simulink model "SYSTEME_ZIGBEE"  (R2016b)
settings: Solver=ode45  StartTime=0.0  StopTime=1E-3  RelTol=1e-3
libraries: dspsrcs4 x6, dsparch4 x5, simulink x3, dspstat3 x2, commsink2 x1, commrandsrc2 x1, commdigbbndcpm2 x1, dspsigops x1
settings Model: DisableUpgradeWarningsForVersion=R2015a  Creator=Yannis  LastModifiedBy=root
settings DataIOCC: LimitDataPoints=on  SaveFormat=Array
settings OptimizationCC: BlockReduction=off  BooleanDataType=off  LifeSpan=inf
settings DebuggingCC: SaveWithParameterizedLinksMsg=none  UnderspecifiedInitializationDetection=Classic  MergeDetectMultiDrivingBlocksExec=none  SignalResolutionControl=TryResolveAllWithWarning  SFUnexpectedBacktrackingDiag=warning  SFNoUnconditionalDefaultTransitionDiag=warning  SFExecutionAtInitializationDiag=none
settings HardwareCC: ProdBitPerPointer=32  ProdBitPerSizeT=32  ProdBitPerPtrDiffT=32  ProdLargestAtomicFloat=None  ProdIntDivRoundTo=Undefined  ProdEndianess=Unspecified  ProdWordSize=32  ProdHWDeviceType=32-bit Generic  TargetBitPerLong=64  TargetBitPerPointer=64  TargetBitPerSizeT=64  TargetBitPerPtrDiffT=64  TargetLongLongMode=on  TargetIntDivRoundTo=Zero  TargetEndianess=LittleEndian  TargetWordSize=64  TargetHWDeviceType=MATLAB Host  ProdEqTarget=off
settings ModelReferenceCC: PropagateSignalLabelsOutOfModel=off
settings GRTTargetCC: TargetLangStandard=C89/C90 (ANSI)  GeneratePreprocessorConditionals=Disable all
settings ConfigComp: CovMetricSettings=dw  CovHtmlReporting=on  CovSaveCumulativeToWorkspaceVar=on  CovSaveSingleToWorkspaceVar=on  CovExternalEMLEnable=off

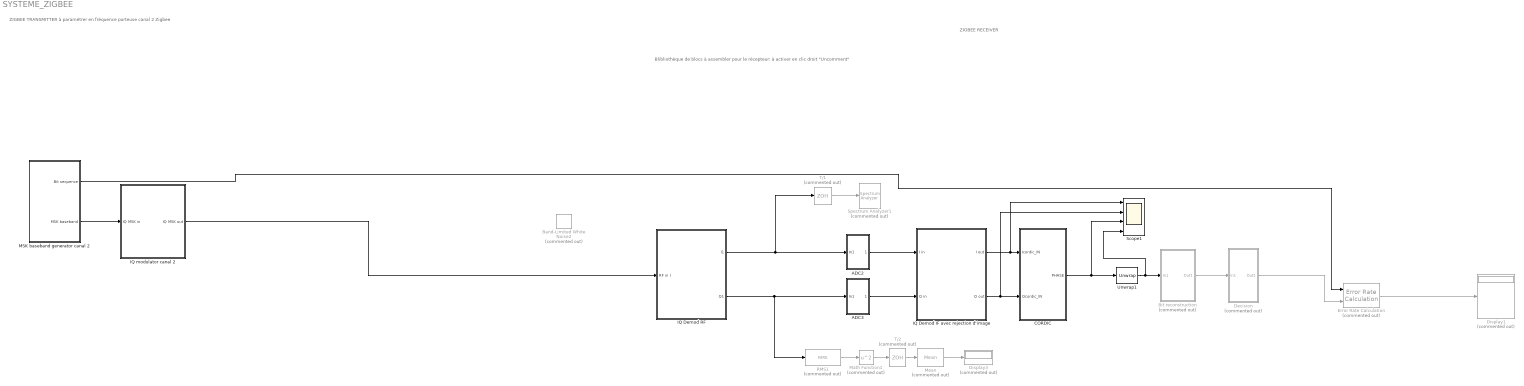
== system SYSTEME_ZIGBEE ==
  note: ZIGBEE RECEIVER
  note: ZIGBEE TRANSMITTER
      | à paramétrer en fréquence porteuse
      | canal 2  Zigbee
  note: Blibliothèque de blocs à assembler pour le récepteur: à activer en clic droit "Uncomment"
  ADC2 : Subsystem
  ADC3 : Subsystem
  Band-Limited White Noise2 : simulink/Sources/Band-Limited White Noise  Commented=on  Cov=[1e-7]  Ts=1e-10  seed=[23341]
  Bit reconstruction : Subsystem  Commented=on
  CORDIC : Subsystem
  Decision : Subsystem  Commented=on
  Display1 : Display  Commented=on
  Display3 : Display  Commented=on
  Error Rate Calculation : commsink2/Error Rate Calculation  Commented=on  N=2  st_delay=1  cp_mode=Entire frame  subframe=[]  PMode=Port  WsName=ErrorVec  RsMode2=off  stop=off  numErr=100  maxBits=1e6
  IQ Demod IF avec rejection d'image : Subsystem  TreatAsAtomicUnit=on
  IQ Demod RF : Subsystem  TreatAsAtomicUnit=on
  IQ modulator canal 2 : Subsystem
  MSK baseband generator canal 2 : Subsystem
  Math Function1 : Math  Commented=on  Operator=square  SaturateOnIntegerOverflow=on
  Mean : dspstat3/Mean  Commented=on  run=on  reset_popup=None  InputProcessing=Columns as channels (frame based)  directionMode=Each column  dimension=1  roiEnable=off  roiType=Rectangles  roiPortion=Entire ROI  roiOutput=Individual statistics for each ROI  roiFlag=off  outputDataTypeStr=Inherit: Same as accumulator  outputLastDataTypeStr=Inherit: Same as accumulator  outputMin=[]  outputMax=[]  roundingMode=Floor  overflowMode=off
  RMS1 : dspstat3/RMS  Commented=on  run=off  directionMode=Entire input  dimension=1  InputProcessing=Columns as channels (frame based)  reset_popup=None
  Scope1 : Scope  NumInputPorts=4
  Spectrum Analyzer1 : SpectrumAnalyzer  Commented=on
  T/1 : ZeroOrderHold  Commented=on  SampleTime=1/(10e6)
  T/2 : ZeroOrderHold  Commented=on  SampleTime=1/(10e6)
  Unwrap1 : dspsigops/Unwrap  tol=pi  InputProcessing=Columns as channels (frame based)  running=off
  wires:
  MSK baseband generator canal 2/2(MSK baseband) -> IQ modulator canal 2/1(IQ MSK in)
  MSK baseband generator canal 2/1(Bit sequence) -> Error Rate Calculation/1
  Error Rate Calculation/1 -> Display1/1
  ADC2/1(Out1) -> IQ Demod IF avec rejection d'image/1("I in ")
  ADC3/1(Out1) -> IQ Demod IF avec rejection d'image/2("Q in ")
  IQ Demod RF/1(I1) -> T/1/1, ADC2/1(In1)
  IQ Demod RF/2("Q1 ") -> RMS1/1, ADC3/1(In1)
  IQ Demod IF avec rejection d'image/1(I out) -> Scope1/1, CORDIC/1(Icordic_IN)
  IQ Demod IF avec rejection d'image/2(Q out) -> Scope1/2, CORDIC/2(Qcordic_IN)
  CORDIC/1(PHASE) -> Scope1/3, Unwrap1/1
  Unwrap1/1 -> Scope1/4, Bit reconstruction/1(In1)
  Bit reconstruction/1(Out1) -> Decision/1(In1)
  T/1/1 -> Spectrum Analyzer1/1
  Decision/1(Out1) -> Error Rate Calculation/2
  RMS1/1 -> Math Function1/1
  Math Function1/1 -> T/2/1
  Mean/1 -> Display3/1
  T/2/1 -> Mean/1
  IQ modulator canal 2/1("IQ MSK out ") -> IQ Demod RF/1(RF in I)

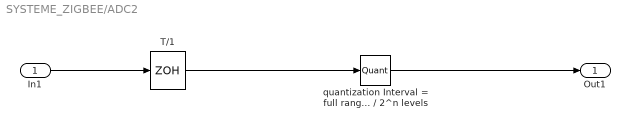
== system SYSTEME_ZIGBEE/ADC2 ==
  In1 : Inport
  T/1 : ZeroOrderHold  SampleTime=1/(10e6)
  quantization Interval = full range (2Volts) / 2^n levels : Quantizer  QuantizationInterval=2/256  LinearizeAsGain=off  SampleTime=1/(10e6)
  Out1 : Outport
  wires:
  In1/1 -> T/1/1
  T/1/1 -> quantization Interval = full range (2Volts) / 2^n levels/1
  quantization Interval = full range (2Volts) / 2^n levels/1 -> Out1/1

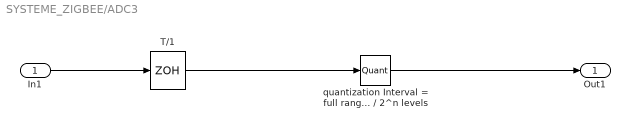
== system SYSTEME_ZIGBEE/ADC3 ==
  In1 : Inport
  T/1 : ZeroOrderHold  SampleTime=1/(10e6)
  quantization Interval = full range (2Volts) / 2^n levels : Quantizer  QuantizationInterval=2/256  LinearizeAsGain=off  SampleTime=1/(10e6)
  Out1 : Outport
  wires:
  In1/1 -> T/1/1
  T/1/1 -> quantization Interval = full range (2Volts) / 2^n levels/1
  quantization Interval = full range (2Volts) / 2^n levels/1 -> Out1/1

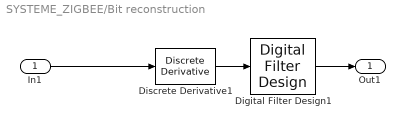
== system SYSTEME_ZIGBEE/Bit reconstruction ==
  In1 : Inport
  Digital Filter Design1 : dsparch4/Digital Filter Design  mwdsp_browser_bugfix_var=off
  Discrete Derivative1 : simulink/Discrete/Discrete Derivative  gainval=1/(10e6)  ICPrevScaledInput=0.0  InputProcessing=Inherited  OutMin=[]  OutMax=[]  OutDataTypeStr=double  OutputDataTypeScalingMode=double  OutDataType=fixdt(1, 16)  OutScaling=2^-10  DoSatur=off
  Out1 : Outport
  wires:
  Discrete Derivative1/1 -> Digital Filter Design1/1
  Digital Filter Design1/1 -> Out1/1
  In1/1 -> Discrete Derivative1/1

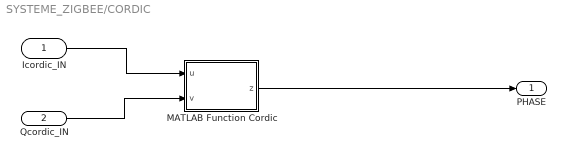
== system SYSTEME_ZIGBEE/CORDIC ==
  Icordic_IN : Inport
  Qcordic_IN : Inport  Port=2
  MATLAB Function Cordic : MATLAB Function  TreatAsAtomicUnit=on
  PHASE : Outport
  wires:
  MATLAB Function Cordic/1(z) -> PHASE/1
  Icordic_IN/1 -> MATLAB Function Cordic/1(u)
  Qcordic_IN/1 -> MATLAB Function Cordic/2(v)

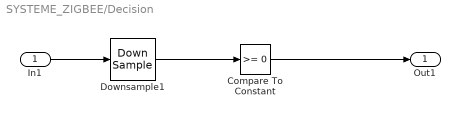
== system SYSTEME_ZIGBEE/Decision ==
  In1 : Inport
  Compare To Constant : simulink/Logic and Bit Operations/Compare To Constant  relop=>=  const=0  OutDataTypeStr=boolean
  Downsample1 : DownSample  N=5  phase=2
  Out1 : Outport
  wires:
  Compare To Constant/1 -> Out1/1
  In1/1 -> Downsample1/1
  Downsample1/1 -> Compare To Constant/1

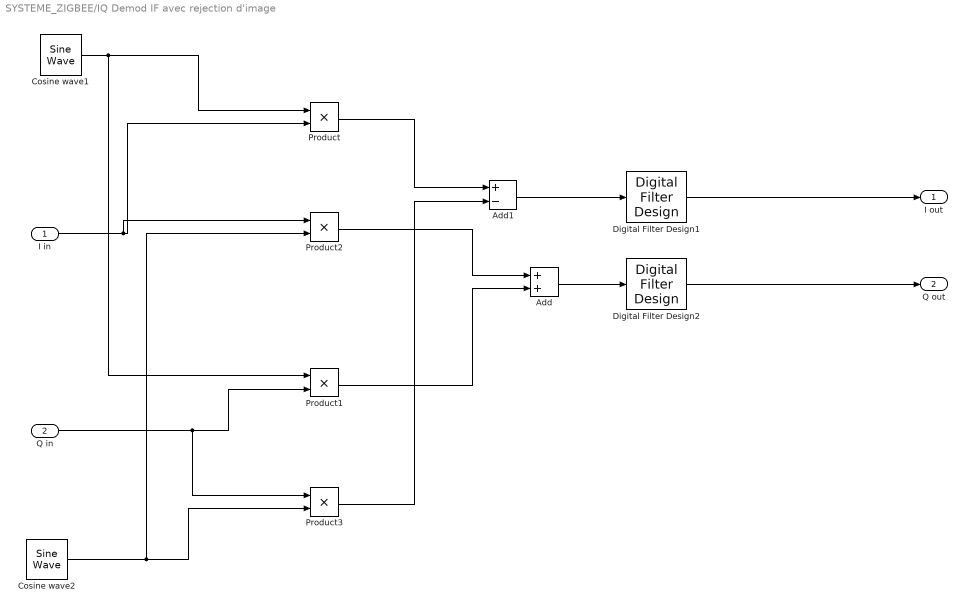
== system SYSTEME_ZIGBEE/IQ Demod IF avec rejection d'image ==
  "I in " : Inport
  "Q in " : Inport  Port=2
  Add : Sum
  Add1 : Sum  Inputs=+-
  Cosine wave1 : dspsrcs4/Sine Wave  Amplitude=1  Frequency=2.5e6  Phase=pi/2  SampleMode=Discrete  OutComplex=Real  CompMethod=Trigonometric fcn  TableSize=Speed  SampleTime=1/(10e6)  SamplesPerFrame=1  ResetState=Restart at time zero  OutputFrames=on  dataType=double  wordLen=16  udDataType=sfix(16)  fracBitsMode=Best precision  numFracBits=15  OutDataTypeStr=double  LastOutDataTypeStr=double
  Cosine wave2 : dspsrcs4/Sine Wave  Amplitude=1  Frequency=2.5e6  Phase=pi  SampleMode=Discrete  OutComplex=Real  CompMethod=Trigonometric fcn  TableSize=Speed  SampleTime=1/(10e6)  SamplesPerFrame=1  ResetState=Restart at time zero  OutputFrames=on  dataType=double  wordLen=16  udDataType=sfix(16)  fracBitsMode=Best precision  numFracBits=15  OutDataTypeStr=double  LastOutDataTypeStr=double
  Digital Filter Design1 : dsparch4/Digital Filter Design  mwdsp_browser_bugfix_var=off
  Digital Filter Design2 : dsparch4/Digital Filter Design  mwdsp_browser_bugfix_var=off
  Product{,1..3} (4 alike) : Product
  I out : Outport
  Q out : Outport  Port=2
  wires:
  Digital Filter Design1/1 -> I out/1
  Digital Filter Design2/1 -> Q out/1
  Cosine wave1/1 -> Product1/1, Product/1
  Cosine wave2/1 -> Product2/2, Product3/2
  "I in "/1 -> Product2/1, Product/2
  "Q in "/1 -> Product3/1, Product1/2
  Product/1 -> Add1/1
  Product3/1 -> Add1/2
  Product2/1 -> Add/1
  Product1/1 -> Add/2
  Add/1 -> Digital Filter Design2/1
  Add1/1 -> Digital Filter Design1/1

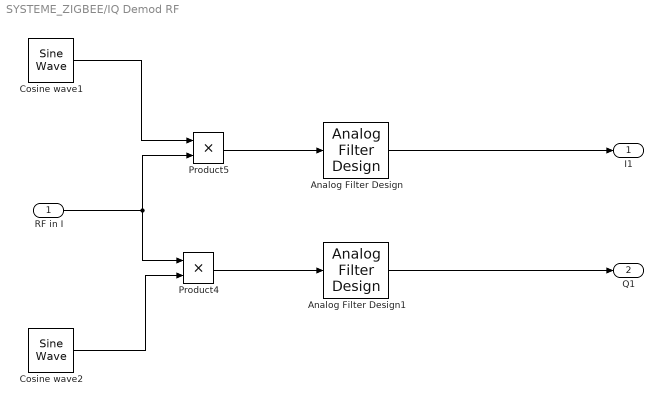
== system SYSTEME_ZIGBEE/IQ Demod RF ==
  RF in I : Inport
  Analog Filter Design : dsparch4/Analog Filter Design  method=Butterworth  filttype=Lowpass  N=8  Wlo=31.4e6  Whi=80  Rp=2  Rs=40
  Analog Filter Design1 : dsparch4/Analog Filter Design  method=Butterworth  filttype=Lowpass  N=8  Wlo=31.4e6  Whi=80  Rp=2  Rs=40
  Cosine wave1 : dspsrcs4/Sine Wave  Amplitude=1  Frequency=2.4075e9  Phase=pi/2  SampleMode=Continuous  OutComplex=Real  CompMethod=Trigonometric fcn  TableSize=Speed  SampleTime=1/(10e6)  SamplesPerFrame=1  ResetState=Restart at time zero  OutputFrames=on  dataType=double  wordLen=16  udDataType=sfix(16)  fracBitsMode=Best precision  numFracBits=15  OutDataTypeStr=double  LastOutDataTypeStr=double
  Cosine wave2 : dspsrcs4/Sine Wave  Amplitude=1  Frequency=2.4075e9  Phase=pi  SampleMode=Continuous  OutComplex=Real  CompMethod=Trigonometric fcn  TableSize=Speed  SampleTime=1/(10e6)  SamplesPerFrame=1  ResetState=Restart at time zero  OutputFrames=on  dataType=double  wordLen=16  udDataType=sfix(16)  fracBitsMode=Best precision  numFracBits=15  OutDataTypeStr=double  LastOutDataTypeStr=double
  Product4 : Product  RndMeth=Zero
  Product5 : Product  RndMeth=Zero
  I1 : Outport
  "Q1 " : Outport  Port=2
  wires:
  RF in I/1 -> Product5/2, Product4/1
  Cosine wave2/1 -> Product4/2
  Cosine wave1/1 -> Product5/1
  Product5/1 -> Analog Filter Design/1
  Product4/1 -> Analog Filter Design1/1
  Analog Filter Design/1 -> I1/1
  Analog Filter Design1/1 -> "Q1 "/1

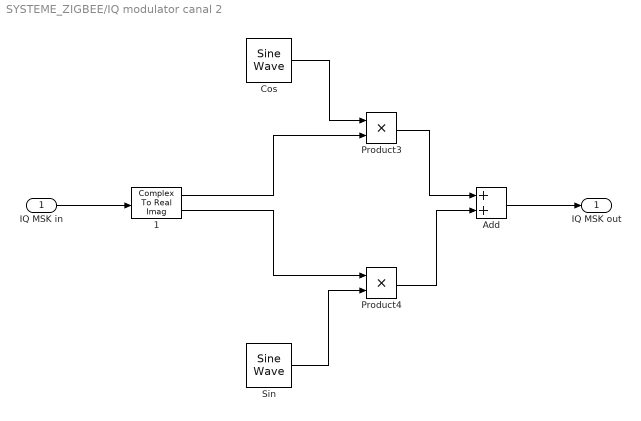
== system SYSTEME_ZIGBEE/IQ modulator canal 2 ==
  IQ MSK in : Inport
  " 1" : ComplexToRealImag
  Add : Sum
  Cos : dspsrcs4/Sine Wave  Amplitude=1  Frequency=2.410e9  Phase=pi/2  SampleMode=Continuous  OutComplex=Real  CompMethod=Trigonometric fcn  TableSize=Speed  SampleTime=1/(8*2.4e9)  SamplesPerFrame=1  ResetState=Restart at time zero  OutputFrames=on  dataType=double  wordLen=16  udDataType=sfix(16)  fracBitsMode=Best precision  numFracBits=15  OutDataTypeStr=double  LastOutDataTypeStr=double
  Product3 : Product  RndMeth=Zero
  Product4 : Product  RndMeth=Zero
  Sin : dspsrcs4/Sine Wave  Amplitude=1  Frequency=2.410E9  Phase=pi  SampleMode=Continuous  OutComplex=Real  CompMethod=Trigonometric fcn  TableSize=Speed  SampleTime=1/(4*2.4e9)  SamplesPerFrame=1  ResetState=Restart at time zero  OutputFrames=on  dataType=double  wordLen=16  udDataType=sfix(16)  fracBitsMode=Best precision  numFracBits=15  OutDataTypeStr=double  LastOutDataTypeStr=double
  "IQ MSK out " : Outport
  wires:
  Add/1 -> "IQ MSK out "/1
  Product4/1 -> Add/2
  " 1"/2 -> Product4/1
  " 1"/1 -> Product3/2
  Sin/1 -> Product4/2
  Product3/1 -> Add/1
  Cos/1 -> Product3/1
  IQ MSK in/1 -> " 1"/1

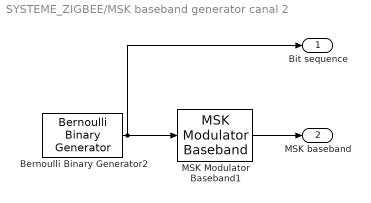
== system SYSTEME_ZIGBEE/MSK baseband generator canal 2 ==
  Bernoulli Binary Generator2 : commrandsrc2/Bernoulli Binary Generator  P=0.5  seed=0  Ts=0.5e-6  frameBased=off  sampPerFrame=1  orient=off  outDataType=boolean
  MSK Modulator Baseband1 : commdigbbndcpm2/MSK Modulator Baseband  inputType=Bit  phaseOffset=0  samplesPerSymbol=1  RateOptions=Enforce single-rate processing  outDataType=double
  Bit sequence : Outport
  MSK baseband : Outport  Port=2
  wires:
  Bernoulli Binary Generator2/1 -> MSK Modulator Baseband1/1, Bit sequence/1
  MSK Modulator Baseband1/1 -> MSK baseband/1

== matlab function SYSTEME_ZIGBEE/CORDIC/MATLAB Function Cordic ==
  data: u input; z output; v input
function z = fcn(u,v)
%#codegen

I0=u;
Q0=v;
I=zeros(1,9);
Q=zeros(1,9);
I(1)=u;
Q(1)=v;
k=0;
z=0;
c1=0;
c2=0;


if I0<0
    if Q0>0
    I(1)=-I0;
    Q(1)=-Q0;
    c1=1;
    end
    if Q0<0
    I(1)=-I0;
    Q(1)=-Q0;
    c2=1;
    end
end

if  I0==0
    if Q0<0;
        z=-pi/2;
    end
    if Q0>0
        z=+pi/2;
    end
end


    
if I(1)>0
    while (k<8)
        if Q(k+1)<0
        Q(k+2)=Q(k+1)+I(k+1)*2^(-k);
        I(k+2)=I(k+1)-Q(k+1)*2^(-k);
        z=z-atan(2^(-(k)));
        end
        if Q(k+1)>0
        Q(k+2)=Q(k+1)-I(k+1)*2^(-k);
        I(k+2)=I(k+1)+Q(k+1)*2^(-k);
        z=z+atan(2^(-k));
        end
        if Q(k+1)==0
        break;
        end
        k=k+1;
    end

end

if c1==1
    z=pi+z;
end

if c2==1
    z=-pi+z;
end

 
end
